simulink model "p2_ipc"  (R2023a)
settings: Solver=ode45  StartTime=0.0  StopTime=200  RelTol=1e-3  EnableMultiTasking=on
settings Model: Creator=Sala S3.5  LastModifiedBy=evely
settings SolverCC: AlgebraicLoopSolver=TrustRegion
settings DataIOCC: LimitDataPoints=on  SaveFormat=Array  ReturnWorkspaceOutputs=off
settings OptimizationCC: LifeSpan=inf
settings DebuggingCC: UnconnectedInputMsg=warning  UnconnectedOutputMsg=warning  UnconnectedLineMsg=warning  SFUnexpectedBacktrackingDiag=warning  SFNoUnconditionalDefaultTransitionDiag=warning  SFExecutionAtInitializationDiag=none  ArithmeticOperatorsInVariantConditions=warning
settings HardwareCC: ProdBitPerPointer=32  ProdBitPerSizeT=32  ProdBitPerPtrDiffT=32  ProdLargestAtomicFloat=None  ProdIntDivRoundTo=Undefined  ProdEndianess=Unspecified  ProdWordSize=32  ProdHWDeviceType=32-bit Generic
settings ModelReferenceCC: PropagateSignalLabelsOutOfModel=off
settings SFSimCC: SimUseLocalCustomCode=off  CustomCodeUndefinedFunction=UseInterfaceOnly
settings RTWCC: RTWUseLocalCustomCode=off
settings CodeAppCC: StateflowObjectComments=on
settings GRTTargetCC: TargetLangStandard=C89/C90 (ANSI)
settings ConfigComp: CovMetricSettings=dw  CovSaveCumulativeToWorkspaceVar=on  CovSaveSingleToWorkspaceVar=on  CovExternalEMLEnable=off

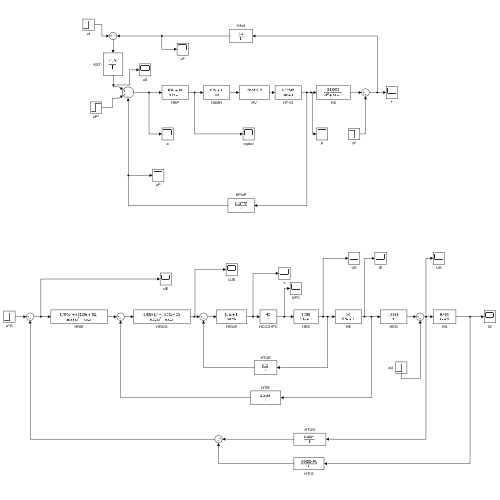
[thumbnail: Simulink's stored preview of the top-level diagram]
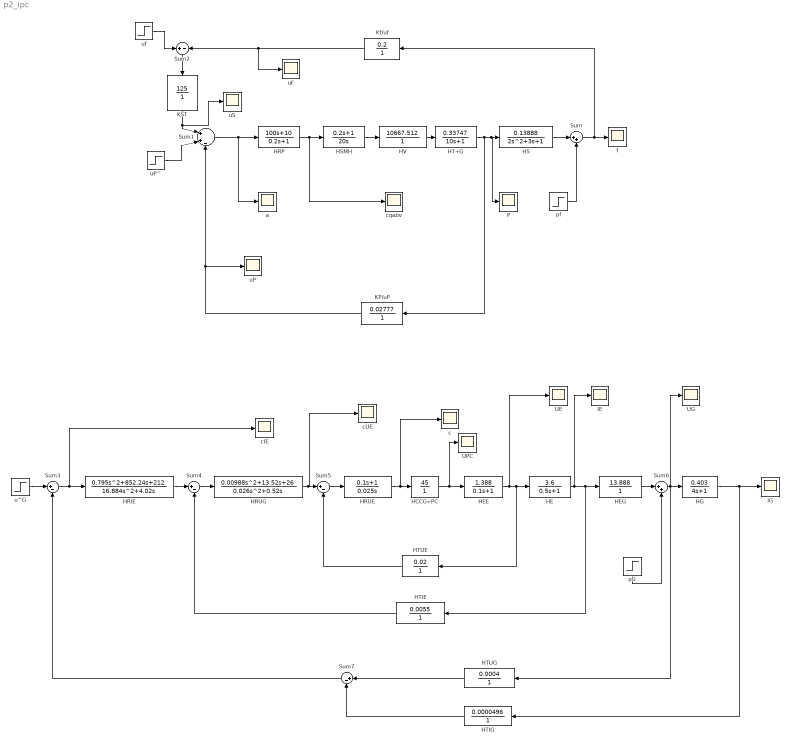
== system p2_ipc ==
  HCCG+PC : TransferFcn  Numerator=[45]  Denominator=[1]
  HE : TransferFcn  Numerator=[3.6]  Denominator=[0.5 1]
  HEE : TransferFcn  Numerator=[1.388]  Denominator=[0.1 1]
  HEG : TransferFcn  Numerator=[13.888]  Denominator=[1]
  HG : TransferFcn  Numerator=[0.403]  Denominator=[4 1]
  HRIE : TransferFcn  Numerator=[0.795 852.24 212]  Denominator=[16.884 4.02 0]
  HRP : TransferFcn  Numerator=[100 10]  Denominator=[0.2 1]
  HRUE : TransferFcn  Numerator=[0.1 1]  Denominator=[0.025 0]
  HRUG : TransferFcn  Numerator=[0.00988 13.52 26]  Denominator=[0.026 0.52 0]
  HS : TransferFcn  Numerator=[0.13888]  Denominator=[2 3 1]
  HSMH : TransferFcn  Numerator=[0.2 1]  Denominator=[20 0]
  HT+G : TransferFcn  Numerator=[0.33747]  Denominator=[10 1]
  HTIE : TransferFcn  Numerator=[0.0055]  Denominator=[1]
  "HTIG " : TransferFcn  Numerator=[0.0000496]  Denominator=[1]
  HTUE : TransferFcn  Numerator=[0.02]  Denominator=[1]
  HTUG : TransferFcn  Numerator=[0.0004]  Denominator=[1]
  HV : TransferFcn  Numerator=[10667.512]  Denominator=[1]
  IE : Scope
  IG : Scope
  KP/uP : TransferFcn  Numerator=[0.02777]  Denominator=[1]
  KST : TransferFcn  Numerator=[125]  Denominator=[1]
  Kf/uf : TransferFcn  Numerator=[0.2]  Denominator=[1]
  P : Scope
  Sum : Sum  Inputs=|++
  Sum1 : Sum  Inputs=|++-
  Sum2 : Sum  Inputs=+-
  Sum{3..5,7} (4 alike) : Sum  Inputs=|+-
  Sum6 : Sum  Inputs=|++
  UE : Scope
  UG : Scope
  UPC : Scope
  a : Scope
  c : Scope
  "cIE " : Scope
  cUE : Scope
  cqabv : Scope
  f : Scope
  pU : Step  SampleTime=0
  pf : Step  Time=150  After=-0.5  SampleTime=0
  uF : Scope
  uP : Scope
  uP^ : Step  Time=0  SampleTime=0
  uS : Scope
  u^G : Step  Time=0  SampleTime=0
  uf : Step  Time=0  SampleTime=0
  wires:
  HRP/1 -> cqabv/1, HSMH/1
  HSMH/1 -> HV/1
  HV/1 -> HT+G/1
  HT+G/1 -> P/1, HS/1, KP/uP/1
  uf/1 -> Sum2/1
  Kf/uf/1 -> uF/1, Sum2/2
  Sum2/1 -> KST/1
  KST/1 -> uS/1, Sum1/1
  uP^/1 -> Sum1/2
  KP/uP/1 -> Sum1/3, uP/1
  Sum1/1 -> a/1, HRP/1
  HS/1 -> Sum/1
  Sum/1 -> Kf/uf/1, f/1
  pf/1 -> Sum/2
  Sum5/1 -> HRUE/1
  HRUE/1 -> HCCG+PC/1, c/1
  HCCG+PC/1 -> HEE/1, UPC/1
  HEE/1 -> HE/1, HTUE/1, UE/1
  Sum6/1 -> HTUG/1, UG/1, HG/1
  HTUE/1 -> Sum5/2
  HTIE/1 -> Sum4/2
  HE/1 -> HEG/1, HTIE/1, IE/1
  HEG/1 -> Sum6/1
  u^G/1 -> Sum3/1
  HG/1 -> "HTIG "/1, IG/1
  HTUG/1 -> Sum7/1
  "HTIG "/1 -> Sum7/2
  Sum7/1 -> Sum3/2
  pU/1 -> Sum6/2
  Sum4/1 -> HRUG/1
  HRUG/1 -> cUE/1, Sum5/1
  Sum3/1 -> HRIE/1, "cIE "/1
  HRIE/1 -> Sum4/1
